simulink model "boostCPM4tester"  (Simulink 7.5)
settings: Solver=ode45  StartTime=0.0  StopTime=0.01  MaxStep=1e-5  RelTol=1e-3
settings Model: Creator=rwe  LastModifiedBy=rwe

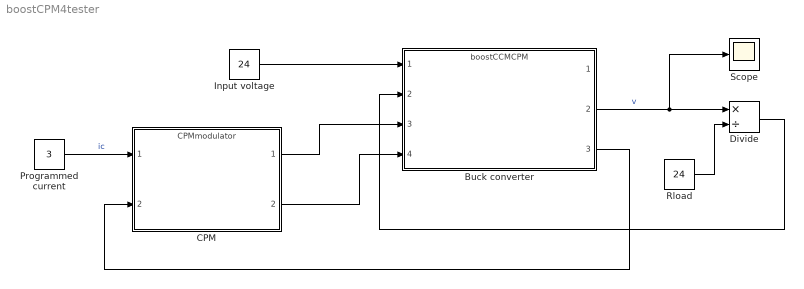
== system boostCPM4tester ==
  Buck converter : ModelReference  ModelNameDialog=boostCCMCPM  SimulationMode=Accelerator  ModelReferenceVersion=1.21  CopyOfModelName=boostCCMCPM
  CPM : ModelReference  ModelNameDialog=CPMmodulator  SimulationMode=Accelerator  ModelReferenceVersion=1.9  CopyOfModelName=CPMmodulator
  Divide : Product  Inputs=*/  OutDataType=fixdt(1, 16)  OutScaling=2^-10
  Input voltage : Constant  Value=24  OutDataType=fixdt(1, 16)  OutScaling=2^0
  Programmed current : Constant  Value=3  OutDataType=fixdt(1, 16)  OutScaling=2^0
  Rload : Constant  Value=24  OutDataType=fixdt(1, 16)  OutScaling=2^0
  Scope : Scope
  wires:
  CPM/1 -> Buck converter/3
  CPM/2 -> Buck converter/4
  Buck converter/3 -> CPM/2
  Buck converter/2 -> Divide/1, Scope/1  "v"
  Rload/1 -> Divide/2
  Divide/1 -> Buck converter/2
  Input voltage/1 -> Buck converter/1
  Programmed current/1 -> CPM/1  "ic"
